simulink model "DSimulator_ur10_3DOF"  (Simulink 10.1)
settings: Solver=ode4  StartTime=0.0  StopTime=120  FixedStep=0.001  RelTol=1e-3  EnableMultiTasking=on
undefined symbols (not defined in the file or in its folder): Dinamic_ur10_3DOF, SimpleRobotPlotROS
settings Model: Creator=E. Dean  LastModifiedBy=tar
settings DataIOCC: LimitDataPoints=on  SignalLoggingSaveFormat=ModelDataLogs
settings OptimizationCC: ExpressionDepthLimit=2147483647
settings DebuggingCC: SolverPrmCheckMsg=warning  FcnCallInpInsideContextMsg=warning  AllowSymbolicDim=off  StateNameClashWarn=warning

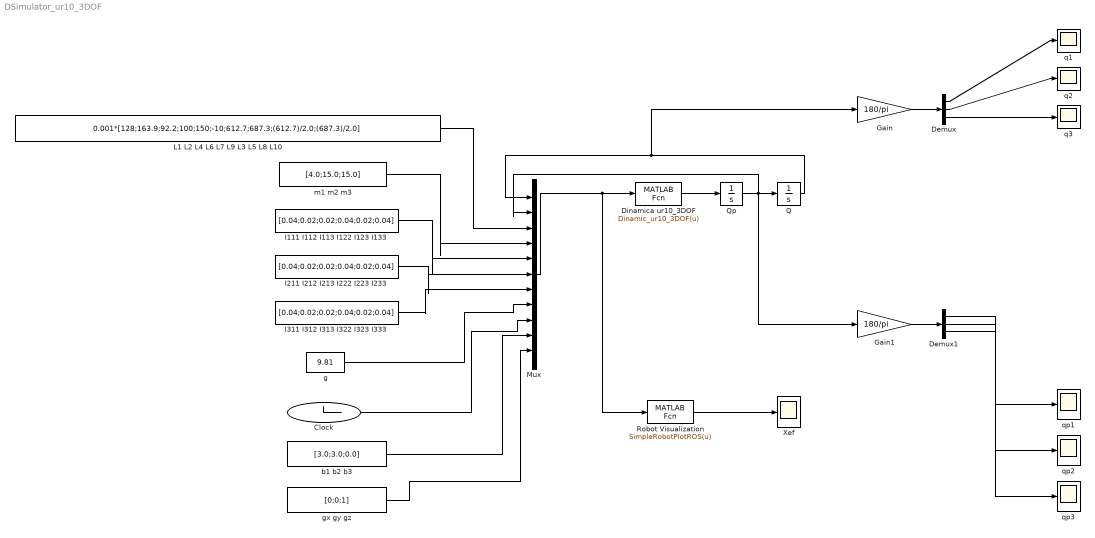
== system DSimulator_ur10_3DOF ==
  Clock : Clock
  Demux : Demux  Outputs=3
  Demux1 : Demux  Outputs=3
  Dinamica ur10_3DOF : MATLABFcn  MATLABFcn=Dinamic_ur10_3DOF(u)  OutputDimensions=3
  Gain : Gain  Gain=180/pi
  Gain1 : Gain  Gain=180/pi
  I111 I112 I113 I122 I123 I133 : Constant  Value=[0.04;0.02;0.02;0.04;0.02;0.04]
  I211 I212 I213 I222 I223 I233 : Constant  Value=[0.04;0.02;0.02;0.04;0.02;0.04]
  I311 I312 I313 I322 I323 I333 : Constant  Value=[0.04;0.02;0.02;0.04;0.02;0.04]
  "L1 L2 L4 L6 L7 L9 L3 L5 L8 L10 " : Constant  Value=0.001*[128;163.9;92.2;100;150;-10;612.7;687.3;(612.7)/2.0;(687.3)/2.0]
  Mux : Mux  Inputs=11
  Q : Integrator  InitialCondition=[pi/4;0;0]
  Qp : Integrator  InitialCondition=[0;0.001;0]
  Robot Visualization : MATLABFcn  MATLABFcn=SimpleRobotPlotROS(u)  OutputDimensions=3
  Xef : Scope
  "b1 b2 b3 " : Constant  Value=[3.0;3.0;0.0]
  g : Constant  Value=9.81
  gx gy gz : Constant  Value=[0;0;1]
  "m1 m2 m3 " : Constant  Value=[4.0;15.0;15.0]
  q1 : Scope
  q2 : Scope
  q3 : Scope
  qp1 : Scope
  qp2 : Scope
  qp3 : Scope
  wires:
  Qp/1 -> Q/1, Gain1/1, Mux/2
  Dinamica ur10_3DOF/1 -> Qp/1
  Q/1 -> Gain/1, Mux/1
  Mux/1 -> Dinamica ur10_3DOF/1, Robot Visualization/1
  Gain/1 -> Demux/1
  Demux/1 -> q1/1
  Demux/2 -> q2/1
  Demux/3 -> q3/1
  Gain1/1 -> Demux1/1
  Demux1/1 -> qp1/1
  Demux1/2 -> qp2/1
  Demux1/3 -> qp3/1
  "L1 L2 L4 L6 L7 L9 L3 L5 L8 L10 "/1 -> Mux/3
  "m1 m2 m3 "/1 -> Mux/4
  I111 I112 I113 I122 I123 I133/1 -> Mux/5
  I211 I212 I213 I222 I223 I233/1 -> Mux/6
  I311 I312 I313 I322 I323 I333/1 -> Mux/7
  g/1 -> Mux/8
  Clock/1 -> Mux/9
  "b1 b2 b3 "/1 -> Mux/10
  gx gy gz/1 -> Mux/11
  Robot Visualization/1 -> Xef/1
